simulink library "demolib"  (R2020a)
settings: Solver=VariableStepAuto  StartTime=0.0  StopTime=10.0  RelTol=1e-3
settings Model: Creator=Anjali123  LastModifiedBy=Anjali123

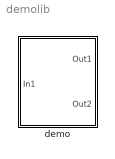
== system demolib ==
  demo : Subsystem  mask{A=40, B=55}
      mask Display: image('$imagefile'); % Use "Edit Image" on toolstrip to change.

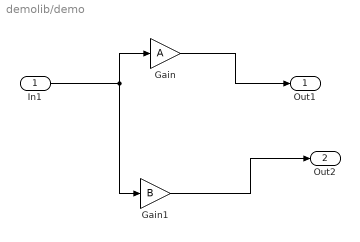
== system demolib/demo ==
  In1 : Inport
  Gain : Gain  Gain=A
  Gain1 : Gain  Gain=B
  Out1 : Outport
  Out2 : Outport  Port=2
  wires:
  Gain1/1 -> Out2/1
  In1/1 -> Gain1/1, Gain/1
  Gain/1 -> Out1/1
